simulink library "powerlib_modelsV2"  (Simulink 6.0)
settings: Solver=ode45  SolverMode=SingleTasking  StartTime=0.0  StopTime=10.0  RelTol=1e-3
undefined symbols (not defined in the file or in its folder): A, Ac, B, Bc, C, Cc, Cs, Current, damp, Dc, Dd, DiscIntNeverNeededParam, dref, dwo, exc, F, fb, gate, GH, GHd, GI, GId, GL, GLd, H, HT, hyd, ib, ib2, io, isfinite, j, K, Kd, Kg, L, Lad, Laq, lim, LIM, Ll, Llfd, Llkd, Llkq1, Llkq2, Llr, Lls, LowerFlux, N, N2, Nb, Nb2, nb_arm, p, Par_HarmoA_pu, Par_HarmoB_pu, Par_Timing_Harmo, Par_Timing_Variation, Par_Vps, Pb ... (+58)
libraries: powerlib_extras x14
(part 4 of 11)

== system powerlib_modelsV2/Continuous/simplified_sync_mach ==
  v : Inport  Port=1  LatchInput=off
  pm : Inport  Port=2  LatchInput=off
  e : Inport  Port=3  LatchInput=off
  1\p : Gain  Gain=1/p  SaturateOnIntegerOverflow=on
  Selector : Selector  Elements=sel  InputPortWidth=3
  Subsystem : Subsystem
  Vt : Subsystem
  Z : Subsystem
      mask Display: disp('Z')
  gen : Subsystem
      mask Display: disp('gen')
  ib : Gain  Gain=ib  SaturateOnIntegerOverflow=on
  mechanics : Subsystem
      mask Display: disp('mec')
  wattmeter : Subsystem  Orientation=left
      mask Display: disp('wattmeter')
  i : Outport  InitialOutput=0
  * : Outport  Port=2  InitialOutput=0
  wires:
  Selector/1 -> i/1
  ib/1 -> Selector/1
  wattmeter/1(Pe) -> mechanics/2(Pe), Subsystem/6(Pe)
  pm/1 -> mechanics/1(Pm)
  e/1 -> gen/2(E)
  mechanics/1(theta_e) -> 1\p/1, gen/1(theta)
  v/1 -> Vt/1(V)
  1\p/1 -> Subsystem/4(theta)
  mechanics/2(wm) -> Subsystem/5(wm)
  Z/1(i) -> ib/1, Subsystem/1(i), wattmeter/1(i)
  gen/1(e) -> Subsystem/3(e), Z/1(e), wattmeter/2(v)  "e"
  Vt/1(Vn) -> gen/3(Vn)
  Vt/2(Vabc) -> Z/2(v), Subsystem/2(v)
  Subsystem/1(*) -> */1

== system powerlib_modelsV2/Continuous/surge_arrester ==
  v : Inport  Port=1  LatchInput=off
  Abs : Abs  SaturateOnIntegerOverflow=on
  Break Alg. Loop : TransferFcn  Denominator="[0.01e-6  1]"
  Product : Product  SaturateOnIntegerOverflow=on  InputSameDT=on
  Sign : Signum  Orientation=down
  Switch1 : Switch  Threshold=ic1  InputSameDT=on
  Switch2 : Switch  Threshold=ic2  InputSameDT=on
  segment1 : Fcn  Expr=p1*(u/uref)^a1
  segment2 : Fcn  Expr=p2*(u/uref)^a2
  segment3 : Fcn  Expr=p3*(u/uref)^a3
  I : Outport  InitialOutput=0
  wires:
  Sign/1 -> Product/2
  Abs/1 -> segment1/1, segment2/1, segment3/1
  segment1/1 -> Switch1/3, Switch1/2
  segment2/1 -> Switch1/1
  Switch2/1 -> Product/1
  Switch1/1 -> Switch2/2, Switch2/3
  segment3/1 -> Switch2/1
  v/1 -> Break Alg. Loop/1
  Break Alg. Loop/1 -> Sign/1, Abs/1
  Product/1 -> I/1

== system powerlib_modelsV2/Continuous/synchronous_machine ==
  v : Inport  Port=1  PortDimensions=2  LatchInput=off
  pm : Inport  Port=2  PortDimensions=1  LatchInput=off
  vf : Inport  Port=3  PortDimensions=1  LatchInput=off
  Delta angle : Subsystem
  Mux : Mux  Inputs=[3,10,6,1,1,1]
  PQ : Subsystem
  Subsystem : Subsystem
  abc2qd : Subsystem
      mask Display: disp('abc/\nqd')
  currents and mutual fluxes : Subsystem
      mask Display: disp('currents\nand\nmutual\nfluxes')
  ia,ib : Selector  Elements=1:2  InputPortWidth=3
  mec : Subsystem
      mask Display: disp('mec')
  phid : Subsystem
      mask Display: disp('phid')
  phifd : Subsystem
      mask Display: disp('phifd')
  phikd : Subsystem
      mask Display: disp('phikd')
  phikq1 : Subsystem
      mask Display: disp('phikq1')
  phikq2 : Subsystem
      mask Display: disp('phikq2')
  phiq : Subsystem
      mask Display: disp('phiq')
  qd2abc : Subsystem
      mask Display: disp('qd/\nabc')
  vkd : Ground
  vkq2 : Ground
  i : Outport  InitialOutput=0
  m : Outport  Port=2  InitialOutput=0
  wires:
  vf/1 -> Subsystem/1(Vf)
  currents and mutual fluxes/2("iq,id,ifd, ikq1,ikq2,ikd, phimq,phimd,vq,vd") -> Mux/2
  vkq2/1 -> phikq2/1(vkq2)
  abc2qd/2(vq) -> phiq/1(vq), Delta angle/1(Vq), currents and mutual fluxes/7(vq), PQ/1(Vq)  "Vq"
  pm/1 -> mec/4(Pm)
  vkd/1 -> phikd/2(vkd)
  phiq/1(phiq) -> phid/2(phiq), mec/3(phiq), currents and mutual fluxes/1(phiq)
  qd2abc/1(is(A)) -> ia,ib/1  "iabc"
  currents and mutual fluxes/1(phimq) -> phiq/4(phimq), phikq2/2(phimq), phikq1/1(phimq)
  qd2abc/2(is(pu)) -> Mux/1
  abc2qd/1(cos,sin) -> qd2abc/1(sin,cos)  "sin,cos"
  currents and mutual fluxes/3(iq,id) -> qd2abc/2(iq,id), mec/1("iq,id "), PQ/3(Iq)  "iq,id"
  ia,ib/1 -> i/1
  phid/1(phid) -> currents and mutual fluxes/3(phid), phiq/3(phid), mec/2(phid)
  abc2qd/3(vd) -> phid/3(vd), Delta angle/2(Vd), currents and mutual fluxes/8(vd), PQ/2(Vd)  "Vd"
  v/1 -> abc2qd/1(v)
  phikd/1(phikd) -> currents and mutual fluxes/6(phikd)
  phifd/1(phifd) -> currents and mutual fluxes/4(phifd)
  phikq1/1(phikq1) -> currents and mutual fluxes/5(phikq1)
  phikq2/1(phikq2) -> currents and mutual fluxes/2(phikq2)
  Subsystem/1(Vkq1) -> phikq1/2(vkq1)
  Subsystem/2(Vfd) -> phifd/1(vfd)
  mec/2(thetae) -> abc2qd/2(theta)
  mec/3(we) -> phiq/2(w), phid/1(w)
  Mux/1 -> m/1
  mec/1(misc) -> Mux/3
  currents and mutual fluxes/4(phimd) -> phid/4(phimd), phifd/2(phimd), phikd/1(phimd)
  PQ/1(Peo) -> Mux/5
  PQ/2(Qeo) -> Mux/6
  Delta angle/1(delta) -> Mux/4

== system powerlib_modelsV2/Continuous/thyristor (logical) ==
  v : Inport  Port=1  LatchInput=off
  g : Inport  Port=2  LatchInput=off
  0 {1..4} (4 alike) : Constant  Value=0
  1/Rsw : Gain  Orientation=down  Gain=1./Rsw  SaturateOnIntegerOverflow=on
  Break Alg. Loop : Subsystem  mask{Nsw=1}
      mask prompts: Nsw "number of switches"
  Constant : Constant  Value=zeros(Nsw,1)
  Data Type  Conversion{1..4} (4 alike) : DataTypeConversion  SaturateOnIntegerOverflow=on  RndMeth=Zero
  Mux : Mux  Inputs=2
  Saturation : Saturate  UpperLimit=inf  LowerLimit=0
  Sum : Sum  Inputs=|++  SaturateOnIntegerOverflow=on  InputSameDT=on
  Switch : Switch  Threshold=0.5  InputSameDT=on
  b5 : RelationalOperator  Operator=>  InputSameDT=on
  b6 : RelationalOperator  Operator=>  InputSameDT=on
  b7 : RelationalOperator  Operator===  InputSameDT=on
  or2 : Logic  Operator=OR
  or3 : Logic  Inputs=3
  vf : Constant  Value=Vf
  i : Outport  InitialOutput=0
  Status : Outport  Port=2  InitialOutput=0
  m : Outport  Port=3  InitialOutput=0
  Vf : Outport  Port=4  InitialOutput=0
  wires:
  Data Type  Conversion4/1 -> or3/3
  Data Type  Conversion3/1 -> or3/2
  g/1 -> Data Type  Conversion4/1  "gate signal"
  0 2/1 -> b6/2
  or3/1 -> or2/2  "Gate = 1 Voltage > 0 Current = 0"
  Mux/1 -> m/1  "measurement signals"
  0 3/1 -> b7/2
  b7/1 -> Data Type  Conversion3/1  "Current = 0"
  or2/1 -> Break Alg. Loop/1(In1)
  Break Alg. Loop/1(Out1) -> Status/1, Switch/2
  0 1/1 -> b5/2
  Constant/1 -> i/1
  v/1 -> b6/1, Sum/1, 1/Rsw/1  "Vak"
  Sum/1 -> Mux/2
  vf/1 -> Sum/2, Vf/1
  b5/1 -> Data Type  Conversion1/1  "Current > 0"
  Data Type  Conversion1/1 -> or2/1
  b6/1 -> Data Type  Conversion2/1  "Voltage > 0"
  Data Type  Conversion2/1 -> or3/1
  Switch/1 -> Saturation/1
  0 4/1 -> Switch/3
  Saturation/1 -> Mux/1, b7/1, b5/1
  1/Rsw/1 -> Switch/1  "Iak"

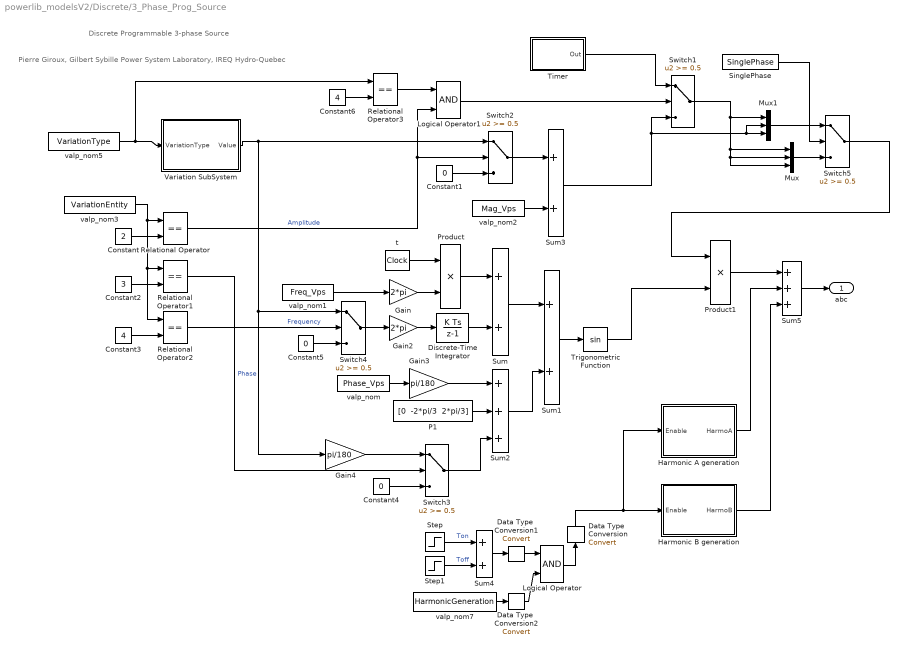
== system powerlib_modelsV2/Discrete/3_Phase_Prog_Source ==
  note: Pierre Giroux, Gilbert Sybille
      | Power System Laboratory, IREQ
      | Hydro-Quebec
  note: Discrete Programmable 3-phase Source
  Constant : Constant  Value=2
  Constant1 : Constant  Value=0
  Constant2 : Constant  Value=3
  Constant3 : Constant  Value=4
  Constant4 : Constant  Value=0
  Constant5 : Constant  Value=0
  Constant6 : Constant  Value=4
  Data Type  Conversion : DataTypeConversion  Orientation=up  SaturateOnIntegerOverflow=on  RndMeth=Zero
  Data Type  Conversion1 : DataTypeConversion  SaturateOnIntegerOverflow=on  RndMeth=Zero
  Data Type  Conversion2 : DataTypeConversion  SaturateOnIntegerOverflow=on  RndMeth=Zero
  Discrete-Time Integrator : DiscreteIntegrator  SampleTime=Ts  SaturateOnIntegerOverflow=on  ICPrevOutput=DiscIntNeverNeededParam  ICPrevScaledInput=DiscIntNeverNeededParam
  Gain : Gain  Gain=2*pi  SaturateOnIntegerOverflow=on
  Gain2 : Gain  Gain=2*pi  SaturateOnIntegerOverflow=on
  Gain3 : Gain  Gain=pi/180  SaturateOnIntegerOverflow=on
  Gain4 : Gain  Gain=pi/180  SaturateOnIntegerOverflow=on
  Harmonic A generation : Subsystem  mask(Harmonic generation){Freq_Vps=Freq_Vps, n_Harmo=n_HarmoA, Mag_Harmo=Mag_HarmoA, Phase_Harmo=Phase_HarmoA, Seq_Harmo=Seq_HarmoA, Ts=Ts}
      mask prompts: Ts "Sample time:"
  Harmonic B generation : Subsystem  mask(Harmonic generation){Freq_Vps=Freq_Vps, n_Harmo=n_HarmoB, Mag_Harmo=Mag_HarmoB, Phase_Harmo=Phase_HarmoB, Seq_Harmo=Seq_HarmoB, Ts=Ts}
      mask prompts: Ts "Sample time:"
  Logical Operator : Logic
  Logical Operator1 : Logic
  Mux : Mux  Inputs=3
  Mux1 : Mux  Inputs=3
  P1 : Constant  Value="[0  -2*pi/3  2*pi/3]"
  Product : Product  SaturateOnIntegerOverflow=on  InputSameDT=on
  Product1 : Product  SaturateOnIntegerOverflow=on  InputSameDT=on
  Relational Operator{,1..3} (4 alike) : RelationalOperator  Operator===  InputSameDT=on
  SinglePhase : Constant  Value=SinglePhase
  Step : Step  Time=Ton_Harmo  SampleTime=Ts
  Step1 : Step  Time=Toff_Harmo  After=-1  SampleTime=Ts
  Sum{,1,3..4} (4 alike) : Sum  SaturateOnIntegerOverflow=on  InputSameDT=on
  Sum2 : Sum  Inputs=+++  SaturateOnIntegerOverflow=on  InputSameDT=on
  Sum5 : Sum  Inputs=+++  SaturateOnIntegerOverflow=on  InputSameDT=on
  Switch{1..5} (5 alike) : Switch  Threshold=0.5  InputSameDT=on
  Timer : Subsystem  mask(Timer){t=Xtime, e=Yampli, Ts=Ts}
      mask prompts: t "Time (s):"; e "Amplitude:"; Ts "Sample time (s)"
      mask help:
      | Generates a signal changing  at specified times.
      |
      | Value of the signal at time zero must  be specified.
      mask init: same as powerlib_modelsV2/Continuous/3_Phase_Prog_Source/Timer
      mask Display: plot( tv(2:end-1), opv(2:end-1) )
  Trigonometric Function : Trigonometry
  Variation SubSystem : Subsystem  mask(Variation Subsystem){VariationStep=VariationStep, VariationRate=VariationRate, VariationFreq=VariationFreq, VariationMag=VariationMag, Ton_Variation=Ton_Variation, Toff_Variation=Toff_Variation, Ts=Ts}
      mask prompts: Ts "Sample time:"
  t : DigitalClock  SampleTime=Ts
  valp_nom : Constant  Value=Phase_Vps
  valp_nom1 : Constant  Value=Freq_Vps
  valp_nom2 : Constant  Value=Mag_Vps
  valp_nom3 : Constant  Value=VariationEntity
  valp_nom5 : Constant  Value=VariationType
  valp_nom7 : Constant  Value=HarmonicGeneration
  abc : Outport  InitialOutput=0
  wires:
  Logical Operator1/1 -> Switch1/2
  Relational Operator3/1 -> Logical Operator1/1
  Switch5/1 -> Product1/1
  Switch1/1 -> Mux1/1, Mux/3, Mux/2, Mux/1
  Mux/1 -> Switch5/3
  SinglePhase/1 -> Switch5/2
  Mux1/1 -> Switch5/1
  Timer/1(Out) -> Switch1/1
  Sum3/1 -> Mux1/2, Mux1/3, Switch1/3
  Constant6/1 -> Relational Operator3/2
  Gain4/1 -> Switch3/1
  Harmonic B generation/1(HarmoB) -> Sum5/3
  Step1/1 -> Sum4/2  "Toff"
  Step/1 -> Sum4/1  "Ton"
  Sum5/1 -> abc/1
  Harmonic A generation/1(HarmoA) -> Sum5/2
  Constant5/1 -> Switch4/3
  Constant3/1 -> Relational Operator2/2
  Constant2/1 -> Relational Operator1/2
  valp_nom3/1 -> Relational Operator1/1, Relational Operator2/1, Relational Operator/1
  Constant/1 -> Relational Operator/2
  Relational Operator2/1 -> Switch4/2  "Frequency"
  Switch4/1 -> Gain2/1
  Variation SubSystem/1(Value) -> Gain4/1, Switch4/1, Switch2/1
  Relational Operator1/1 -> Switch3/2  "Phase"
  Constant4/1 -> Switch3/3
  Switch3/1 -> Sum2/3
  valp_nom5/1 -> Relational Operator3/1, Variation SubSystem/1(VariationType)
  Relational Operator/1 -> Logical Operator1/2, Switch2/2  "Amplitude"
  valp_nom2/1 -> Sum3/2
  Sum2/1 -> Sum1/2
  Constant1/1 -> Switch2/3
  Switch2/1 -> Sum3/1
  Product1/1 -> Sum5/1
  valp_nom1/1 -> Gain/1
  valp_nom/1 -> Gain3/1
  Gain3/1 -> Sum2/1
  Trigonometric Function/1 -> Product1/2
  P1/1 -> Sum2/2
  Discrete-Time Integrator/1 -> Sum/2
  Gain2/1 -> Discrete-Time Integrator/1
  Sum1/1 -> Trigonometric Function/1
  Sum/1 -> Sum1/1
  t/1 -> Product/1
  Gain/1 -> Product/2
  Product/1 -> Sum/1
  Logical Operator/1 -> Data Type  Conversion/1
  Data Type  Conversion/1 -> Harmonic A generation/1(Enable), Harmonic B generation/1(Enable)
  Sum4/1 -> Data Type  Conversion1/1
  Data Type  Conversion1/1 -> Logical Operator/1
  valp_nom7/1 -> Data Type  Conversion2/1
  Data Type  Conversion2/1 -> Logical Operator/2

== system powerlib_modelsV2/Discrete/3_phase_source ==
  Constant : Constant  Value=complex(A*cos(P*pi/180),A*sin(P*pi/180))
  Constant1 : Constant  Value=complex(A*cos((P-120)*pi/180),A*sin((P-120)*pi/180))
  Constant2 : Constant  Value=complex(A*cos((P+120)*pi/180),A*sin((P+120)*pi/180))
  Mux : Mux  Inputs=6
  Sine Wave : Sin  Amplitude=A  Frequency=2*pi*F  Phase=P*pi/180  SampleTime=Ts
  Sine Wave1 : Sin  Amplitude=A  Frequency=2*pi*F  Phase=(P-120)*pi/180  SampleTime=Ts
  Sine Wave2 : Sin  Amplitude=A  Frequency=2*pi*F  Phase=(P+120)*pi/180  SampleTime=Ts
  Out1 : Outport
  wires:
  Mux/1 -> Out1/1
  Constant2/1 -> Mux/6
  Sine Wave2/1 -> Mux/5
  Constant1/1 -> Mux/4
  Sine Wave1/1 -> Mux/3
  Sine Wave/1 -> Mux/1
  Constant/1 -> Mux/2

== system powerlib_modelsV2/Discrete/Dynamic_Load ==
  v : Inport  Port=1  PortDimensions=2  LatchInput=off
  PQ : Inport  Port=2  PortDimensions=2  LatchInput=off
  Complex to Real-Imag : ComplexToRealImag  Orientation=left
  Demux : Demux  Outputs=2
  Discrete 3-phase PLL : Subsystem  mask(Discrete 3-phase PLL){Par_Init=[Pha_V0  fnom], ParK=[60 1400], Ts=Ts}
      mask prompts: Par_Init "Initial inputs:[ Phase(degrees)   Frequency(Hz) ]"; ParK "Regulator gains [ Kp  Ki ]"; Ts "Sample time:"
      mask init:
      | Kp=ParK(1);
      | Ki=ParK(2);
      | Phase_Init=Par_Init(1);
      | Finit=Par_Init(2);
  Discrete Variable Frequency Mean value : powerlib_extras/Discrete Measurements/Discrete Variable Frequency Mean value  Finit=fnom  Fmin=45  Vinit=Mag_V0  Ts=Ts
  Discrete Variable Frequency Mean value1 : powerlib_extras/Discrete Measurements/Discrete Variable Frequency Mean value  Finit=fnom  Fmin=45  Vinit=0  Ts=Ts
  Ground : Ground  Orientation=left
  Mux1 : Mux  Orientation=left  Inputs=3
  Positive Sequence  current : Subsystem
  Real-Imag to Complex : RealImagToComplex
  Real-Imag to Complex1 : RealImagToComplex
  Selector : Selector  Orientation=left  Elements=1:2  InputPortWidth=3
  Unit Delay2 : UnitDelay  Orientation=left  X0=I1_init*exp(-j*Pha_V0*pi/180)  SampleTime=Ts
  V> pu : Gain  Gain=1/Vbase  SaturateOnIntegerOverflow=on
  dq0_to_abc Transformation : powerlib_extras/Measurements/dq0_to_abc Transformation  Orientation=left
  i : Outport  Orientation=left
  m : Outport  Port=2
  wires:
  dq0_to_abc Transformation/1 -> Selector/1
  Selector/1 -> i/1
  v/1 -> V> pu/1
  V> pu/1 -> Discrete 3-phase PLL/1(Vab_bc (pu))
  Real-Imag to Complex/1 -> Positive Sequence  current/1(V1(pu))
  Mux1/1 -> dq0_to_abc Transformation/1
  Unit Delay2/1 -> Complex to Real-Imag/1
  Discrete 3-phase PLL/3(Vq) -> Discrete Variable Frequency Mean value1/2
  Ground/1 -> Mux1/3
  Discrete Variable Frequency Mean value/1 -> Real-Imag to Complex/1
  Discrete Variable Frequency Mean value1/1 -> Real-Imag to Complex/2
  Positive Sequence  current/1(I1(A)) -> Unit Delay2/1
  Complex to Real-Imag/1 -> Mux1/1
  Complex to Real-Imag/2 -> Mux1/2
  Discrete 3-phase PLL/2(Vd) -> Discrete Variable Frequency Mean value/2
  Discrete 3-phase PLL/4(sin_cos) -> dq0_to_abc Transformation/2
  Discrete 3-phase PLL/1(Freq) -> Discrete Variable Frequency Mean value/1, Discrete Variable Frequency Mean value1/1
  PQ/1 -> Demux/1
  Demux/1 -> Real-Imag to Complex1/1
  Demux/2 -> Real-Imag to Complex1/2
  Real-Imag to Complex1/1 -> Positive Sequence  current/2(S_ext)
  Positive Sequence  current/2(VPQ) -> m/1

== system powerlib_modelsV2/Discrete/Excitation_System ==
  vref : Inport  Port=1  LatchInput=off
  vd : Inport  Port=2  LatchInput=off
  vq : Inport  Port=3  LatchInput=off
  vstab : Inport  Port=4  LatchInput=off
  Damping kf.s / (tf.s +1) : Subsystem  Orientation=left
  Exciter  1 / (te.s + ke) : Subsystem
  Lead Lag Compensator tc.s+1 / tb.s+1 : powerlib_extras/Discrete  Control Blocks/Discrete Lead-Lag  T1=tc  T2=tb  V_Init=ke*v0(2)/ka  Ts=Ts
  Low Pass Filter 1 / (tr.s +1) (with IC) : powerlib_extras/Discrete  Control Blocks/Discrete 1st-Order Discrete Filter  FilterType=Lowpass  Tc=tr  Ts=Ts  Initialize=on  Vac_Init=[0 0 60]  Vdc_Init=v0(1)  PlotResponse=off  param1=[1 500 0.1]
  Main Regulator ka / (ta.s +1) : Subsystem
  Mux : Mux  Inputs=2
  Positive Seqence Voltage : Fcn  Expr=sqrt(u(1)^2 + u(2)^2)
  Sum : Sum  Inputs=++-+-  SaturateOnIntegerOverflow=on  InputSameDT=on
  Unit Delay1 : UnitDelay  Orientation=left  SampleTime=Ts
  Unit Delay2 : UnitDelay  X0=v0(2)  SampleTime=Ts
  Vf0 \ ka : Constant  Value=v0(2)/ka
  proportionnal saturation : Subsystem
  Vf : Outport  InitialOutput=0
  wires:
  Unit Delay2/1 -> Vf/1
  Unit Delay1/1 -> Sum/5
  proportionnal saturation/1(Ef) -> Exciter  1 / (te.s + ke)/1(In)
  Lead Lag Compensator tc.s+1 / tb.s+1/1 -> Main Regulator ka / (ta.s +1)/1(In)
  Sum/1 -> Lead Lag Compensator tc.s+1 / tb.s+1/1
  Positive Seqence Voltage/1 -> Low Pass Filter 1 / (tr.s +1) (with IC)/1
  vq/1 -> Mux/2
  vd/1 -> Mux/1
  Mux/1 -> Positive Seqence Voltage/1
  vref/1 -> Sum/1
  vstab/1 -> Sum/4
  Low Pass Filter 1 / (tr.s +1) (with IC)/1 -> proportionnal saturation/2(Vtf), Sum/3
  Vf0 \ ka/1 -> Sum/2
  Main Regulator ka / (ta.s +1)/1(Out) -> proportionnal saturation/1(Efd)
  Damping kf.s / (tf.s +1)/1(Out) -> Unit Delay1/1
  Exciter  1 / (te.s + ke)/1(Out) -> Unit Delay2/1, Damping kf.s / (tf.s +1)/1(In)

== system powerlib_modelsV2/Discrete/GTO-IGBT Bridge ==
  note: *
      | *
      | ||
      | ||
      | *
      | *
      | *
      | ||
      | ||
      | *
      | *
  note: 1
  note: 2
  note: +
  note: -
  note: *
      | *
      | ||
      | ||
      | *
      | *
      | *
      | ||
      | ||
      | *
      | *
  note: 3
  note: 4
  note: ***********************************************
  note: Vcc
  note: A
  note: B
  note: *
      | *
      | ||
      | ||
      | *
      | *
      | *
      | ||
      | ||
      | *
      | *
  note: C
  note: ***********************************************
  note: 5
  note: 6
  note: GTO:
      |  tail current can be turned off by specifying Tf=0 and Tt=0
  note: Diode Logic :
      | 1) Diodes are blocked when complementary GTOs are switched on
      | 2) When no snubber capacitances are used (Cs=inf), diodes are triggered
      | when complementary GTOs are swithed off
  v : Inport  Port=1  LatchInput=off
  g : Inport  Port=2  LatchInput=off
  1/Rsw : Gain  Orientation=up  Gain=1./Rsw  SaturateOnIntegerOverflow=on
  2 : Constant  Value=Tf>0 | Tt>0
  Constant1 : Constant  Value=0
  Data Type  Conversion{2..5} (4 alike) : DataTypeConversion  SaturateOnIntegerOverflow=on  RndMeth=Zero
  Diode Logic : Subsystem
  GTO Logic : Subsystem
  G_D : Logic  Operator=OR
  Gain : Gain  Orientation=up  Gain=-1  SaturateOnIntegerOverflow=on
  Product : Product  SaturateOnIntegerOverflow=on  InputSameDT=on
  Relational Operator : RelationalOperator  InputSameDT=on
  Tail discrete : Subsystem  TreatAsAtomicUnit=on  mask(Gto tail current){}
  Unit Delay : UnitDelay  SampleTime=Ts
  Unit Delay3 : UnitDelay  SampleTime=Ts
  "Vf " : Subsystem
  iTail : Outport
  status : Outport  Port=2
  Vf : Outport  Port=3
  wires:
  2/1 -> Tail discrete/Enable
  Relational Operator/1 -> Diode Logic/2(Ipos), Data Type  Conversion3/1
  Constant1/1 -> Relational Operator/2
  Unit Delay/1 -> Tail discrete/1(Iak)
  Gain/1 -> Diode Logic/1(Vak)
  Product/1 -> Unit Delay/1  "IGTO"
  Tail discrete/1(itail) -> iTail/1
  1/Rsw/1 -> Product/2, Relational Operator/1
  v/1 -> Gain/1, GTO Logic/1(Vak), 1/Rsw/1
  "Vf "/1(Vf) -> Vf/1
  GTO Logic/1(status) -> G_D/2, Diode Logic/3(G), "Vf "/1(status_GTO)
  Data Type  Conversion3/1 -> Product/1
  g/1 -> Data Type  Conversion4/1
  Data Type  Conversion4/1 -> Tail discrete/2(switch), GTO Logic/2(G)
  Diode Logic/1(status) -> Data Type  Conversion5/1
  Data Type  Conversion5/1 -> G_D/1
  Unit Delay3/1 -> status/1
  G_D/1 -> Data Type  Conversion2/1
  Data Type  Conversion2/1 -> Unit Delay3/1

== system powerlib_modelsV2/Discrete/HTG ==
  wref : Inport  Port=1  LatchInput=off
  Pref : Inport  Port=2  LatchInput=off
  we : Inport  Port=3  LatchInput=off
  Pe : Inport  Port=4  LatchInput=off
  dw : Inport  Port=5  LatchInput=off
  Constant1 : Constant  Orientation=left  Value=dref
  Discrete PID Controller : Subsystem  AncestorBlock=|  mask(Discrete PID Controller){Kp=kp, Ki=ki, Kd=kd, TcD=td, Par_Limits=[1e6 -1e6], Init=go, Ts=Ts}
      | powerlib_extras/Discrete 
      | Control Blocks/Discrete
      | PID Controller
      mask prompts: Kp "Proportional gain (Kp):"; Ki "Integral gain (Ki):"; Kd "Derivative gain (Kd):"; TcD "Time constant for derivative (s):"; Par_Limits "Output limits: [ Upper   Lower ]"; Init "Output initial value:"; Ts "Sample time:"
      mask help: This block implements a discrete PID controller.
      mask init:
      | UpperLimit=Par_Limits(1);
      | LowerLimit=Par_Limits(2);
      mask Display: disp('PID');
  Sum : Sum  Inputs=+-  SaturateOnIntegerOverflow=on  InputSameDT=on
  Sum1 : Sum  Inputs=+-  SaturateOnIntegerOverflow=on  InputSameDT=on
  Sum5 : Sum  Inputs=-+  SaturateOnIntegerOverflow=on  InputSameDT=on
  Switch : Switch  Orientation=left  Threshold=0.5  InputSameDT=on
  permanent droop : Gain  Orientation=left  Gain=Rp  SaturateOnIntegerOverflow=on
  servo-motor : Subsystem
      mask Display: disp('servo-\nmotor')
  turbine : Subsystem
      mask Display: disp('hydraulic\nturbine')
  Pm : Outport  InitialOutput=0
  gate : Outport  Port=2  InitialOutput=0
  wires:
  Constant1/1 -> Switch/2
  Switch/1 -> permanent droop/1
  Pe/1 -> Sum5/2
  Pref/1 -> Sum5/1
  Sum1/1 -> Discrete PID Controller/1(Error)
  permanent droop/1 -> Sum1/2
  Sum/1 -> Sum1/1
  Discrete PID Controller/1(Out) -> servo-motor/1(regulator's output)
  wref/1 -> Sum/1
  we/1 -> Sum/2
  Sum5/1 -> Switch/3
  servo-motor/1(gate opening) -> turbine/2(gate opening), gate/1, Switch/1
  dw/1 -> turbine/1(dw)
  turbine/1(Pm) -> Pm/1

== system powerlib_modelsV2/Discrete/Impedance Measurement ==
  v : Inport  Port=1  LatchInput=off
  Ground : Ground
  Terminator : Terminator
  i : Outport  InitialOutput=0
  wires:
  v/1 -> Terminator/1
  Ground/1 -> i/1

== system powerlib_modelsV2/Discrete/MBPSS ==
  note: (for simplified
      | settings only)
  note: Low and intermediate speed deviation is based on the internal voltage phasors while
      | the high frequency speed deviation  is based on the electrical power.
  note: Note: Speed deviation is derived from the machine positive-sequence terminal voltages and currents.
  note: (IEEE Type PSS4b)
  note: Discrete Multi-band Power System Stabilizer
  note: Innocent Kamwa, Robert Grondin
      | IREQ, Hydro-Quebec
  dw : Inport  Port=1  LatchInput=off
  Constant : Constant  Value=Detailed
  Discrete Lead-Lag1 : Subsystem  mask(Discrete Lead-Lag Compensator){values=[TL1 TL2 KL11], Ts=Ts}
      mask prompts: values "Coefficients values: [ T1 T2 K1 ]"; Ts "Sample time (s):"
      mask help:
      | This block implements a discrete lead-lag compensator:
      |
      |          T1.s + K1
      | H(s)= --------
      |            T2.s + 1
      mask init:
      | numc=[values(1) values(3)];
      | denc=[values(2) 1];
      | [Ac,Bc,Cc,Dc]=tf2ss(numc,denc);
      | %
      | %  Conversion to discrete transfer function
      | nstates = size(Ac,1);
      | invexp = inv(eye(nstates) - (Ts/2)*Ac);
      | Ad = invexp*(eye(nstates) + (Ts/2)*Ac);
      | Bd = invexp*Bc;
      | Cd = Cc*invexp*Ts;
      | Dd = Cc*invexp*Bc*(Ts/2) + Dc;
      | %
      | if values(1)==0 & values(2)==0, Dd=1; end
      mask Display: disp('TL1.s+KL11\n---\nTL2.s+1')
  Discrete Lead-Lag2 : Subsystem  mask(Discrete Lead-Lag Compensator){values=[TL7 TL8 KL17], Ts=Ts}
      mask prompts: values "Coefficients values: [ T1 T2 K1 ]"; Ts "Sample time (s):"
      mask help:
      | This block implements a discrete lead-lag compensator:
      |
      |          T1.s + K1
      | H(s)= --------
      |            T2.s + 1
      mask init: same as powerlib_modelsV2/Discrete/MBPSS/Discrete Lead-Lag1
      mask Display: disp('TL7.s+KL17\n---\nTL8.s+1')
  Discrete Lead-Lag3 : Subsystem  mask(Discrete Lead-Lag Compensator){values=[TI1 TI2 KI11], Ts=Ts}
      mask prompts: values "Coefficients values: [ T1 T2 K1 ]"; Ts "Sample time (s):"
      mask help:
      | This block implements a discrete lead-lag compensator:
      |
      |          T1.s + K1
      | H(s)= --------
      |            T2.s + 1
      mask init: same as powerlib_modelsV2/Discrete/MBPSS/Discrete Lead-Lag1
      mask Display: disp('TI1.s+KI11\n---\nTI2.s+1')
  Discrete Lead-Lag4 : Subsystem  mask(Discrete Lead-Lag Compensator){values=[TI7 TI8 KI17], Ts=Ts}
      mask prompts: values "Coefficients values: [ T1 T2 K1 ]"; Ts "Sample time (s):"
      mask help:
      | This block implements a discrete lead-lag compensator:
      |
      |          T1.s + K1
      | H(s)= --------
      |            T2.s + 1
      mask init: same as powerlib_modelsV2/Discrete/MBPSS/Discrete Lead-Lag1
      mask Display: disp('TI7.s+KI17\n---\nTI8.s+1')
  Discrete Lead-Lag5 : Subsystem  mask(Discrete Lead-Lag Compensator){values=[TH1 TH2 KH11], Ts=Ts}
      mask prompts: values "Coefficients values: [ T1 T2 K1 ]"; Ts "Sample time (s):"
      mask help:
      | This block implements a discrete lead-lag compensator:
      |
      |          T1.s + K1
      | H(s)= --------
      |            T2.s + 1
      mask init: same as powerlib_modelsV2/Discrete/MBPSS/Discrete Lead-Lag1
      mask Display: disp('TH1.s+KH11\n---\nTH2.s+1')
  Discrete Lead-Lag6 : Subsystem  mask(Discrete Lead-Lag Compensator){values=[TH7 TH8 KH17], Ts=Ts}
      mask prompts: values "Coefficients values: [ T1 T2 K1 ]"; Ts "Sample time (s):"
      mask help:
      | This block implements a discrete lead-lag compensator:
      |
      |          T1.s + K1
      | H(s)= --------
      |            T2.s + 1
      mask init: same as powerlib_modelsV2/Discrete/MBPSS/Discrete Lead-Lag1
      mask Display: disp('TH7.s+KH17\n---\nTH8.s+1')
  Gain : Gain  Gain=KL  SaturateOnIntegerOverflow=on
  Gain1 : Gain  Gain=KI  SaturateOnIntegerOverflow=on
  Gain2 : Gain  Gain=KH  SaturateOnIntegerOverflow=on
  Gain3 : Gain  Gain=KL1  SaturateOnIntegerOverflow=on
  Gain4 : Gain  Gain=KL2  SaturateOnIntegerOverflow=on
  Gain5 : Gain  Gain=KI1  SaturateOnIntegerOverflow=on
  Gain6 : Gain  Gain=KI2  SaturateOnIntegerOverflow=on
  Gain7 : Gain  Gain=KH1  SaturateOnIntegerOverflow=on
  Gain8 : Gain  Gain=KH2  SaturateOnIntegerOverflow=on
  Gain9 : Gain  Gain=Kg  SaturateOnIntegerOverflow=on
  HF speed sensor : Subsystem  mask(discrete state-space model (PSB)){numc=[80 0 0], denc=[1 82 161 80], Ts=Ts}
      mask prompts: numc "Numerator:"; denc "Denominator:"; Ts "Sample time (s):"
      mask help: This block implements a discrete state-space model based on the coefficients of a continuous transfer function. Coefficients must be given in descending power of s.
      mask init:
      | [Ac,Bc,Cc,Dc]=tf2ss(numc,denc);
      | %
      | %  Conversion to discrete transfer function
      | nstates = size(Ac,1);
      | invexp = inv(eye(nstates) - (Ts/2)*Ac);
      | Ad = invexp*(eye(nstates) + (Ts/2)*Ac);
      | Bd = invexp*Bc;
      | Cd = Cc*invexp*Ts;
      | Dd = Cc*invexp*Bc*(Ts/2) + Dc;
      mask Display: disp('Discrete\nState-space\nModel')
  LF and IF speed sensor : Subsystem  mask(discrete state-space model (PSB)){numc=[-1.759e-3 1], denc=[1.2739e-4 1.7823e-2 1], Ts=Ts}
      mask prompts: numc "Numerator:"; denc "Denominator:"; Ts "Sample time (s):"
      mask help: This block implements a discrete state-space model based on the coefficients of a continuous transfer function. Coefficients must be given in descending power of s.
      mask init: same as powerlib_modelsV2/Discrete/MBPSS/HF speed sensor
      mask Display: disp('Discrete\nState-space\nModel')
  "Limiteur BF " : Saturate  UpperLimit=LIM_VL  LowerLimit=-LIM_VL
  Limiteur HF : Saturate  UpperLimit=LIM_VH  LowerLimit=-LIM_VH
  "Limiteur IF " : Saturate  UpperLimit=LIM_VI  LowerLimit=-LIM_VI
  Limiteur VS : Saturate  UpperLimit=LIM_VS  LowerLimit=-LIM_VS
  Sum : Sum  Inputs=+-  SaturateOnIntegerOverflow=on  InputSameDT=on
  Sum1 : Sum  Inputs=+++  SaturateOnIntegerOverflow=on  InputSameDT=on
  Sum2 : Sum  Inputs=+-  SaturateOnIntegerOverflow=on  InputSameDT=on
  Sum3 : Sum  Inputs=+-  SaturateOnIntegerOverflow=on  InputSameDT=on
  Transfer function for detailed model (HF) : Subsystem
  Transfer function for detailed model (IF) : Subsystem
  Transfer function for detailed model (LF) : Subsystem
  VS : Outport  InitialOutput=0
  wires:
  Gain9/1 -> Limiteur VS/1
  Constant/1 -> Transfer function for detailed model (HF)/1(On), Transfer function for detailed model (IF)/1(On), Transfer function for detailed model (LF)/1(On)
  Limiteur VS/1 -> VS/1
  Sum1/1 -> Gain9/1
  Limiteur HF/1 -> Sum1/3
  "Limiteur IF "/1 -> Sum1/2
  "Limiteur BF "/1 -> Sum1/1
  Sum3/1 -> Gain2/1
  Transfer function for detailed model (HF)/2(LFneg) -> Sum3/2
  Transfer function for detailed model (HF)/1(HFpos) -> Sum3/1
  Discrete Lead-Lag6/1(Out1) -> Transfer function for detailed model (HF)/3("HFneg ")
  Discrete Lead-Lag5/1(Out1) -> Transfer function for detailed model (HF)/2("HFpos ")
  Sum2/1 -> Gain1/1
  Discrete Lead-Lag4/1(Out1) -> Transfer function for detailed model (IF)/3("IFneg ")
  Discrete Lead-Lag3/1(Out1) -> Transfer function for detailed model (IF)/2("IFpos ")
  Transfer function for detailed model (IF)/2(IFneg) -> Sum2/2
  Transfer function for detailed model (IF)/1(IFpos) -> Sum2/1
  Discrete Lead-Lag2/1(Out1) -> Transfer function for detailed model (LF)/3("LFneg ")
  Discrete Lead-Lag1/1(Out1) -> Transfer function for detailed model (LF)/2("LFpos ")
  Transfer function for detailed model (LF)/2(LFneg) -> Sum/2
  Transfer function for detailed model (LF)/1(LFpos) -> Sum/1
  Sum/1 -> Gain/1
  Gain/1 -> "Limiteur BF "/1
  Gain1/1 -> "Limiteur IF "/1
  Gain2/1 -> Limiteur HF/1
  Gain3/1 -> Discrete Lead-Lag1/1(In1)
  Gain4/1 -> Discrete Lead-Lag2/1(In1)
  Gain5/1 -> Discrete Lead-Lag3/1(In1)
  Gain6/1 -> Discrete Lead-Lag4/1(In1)
  Gain7/1 -> Discrete Lead-Lag5/1(In1)
  Gain8/1 -> Discrete Lead-Lag6/1(In1)
  LF and IF speed sensor/1(Out) -> Gain3/1, Gain4/1, Gain5/1, Gain6/1
  HF speed sensor/1(Out) -> Gain8/1, Gain7/1
  dw/1 -> HF speed sensor/1(In), LF and IF speed sensor/1(In)

== system powerlib_modelsV2/Discrete/PM_synchronous_machine ==
  v : Inport  Port=1  LatchInput=off
  Tm : Inport  Port=2  LatchInput=off
  Mux : Mux  Inputs=[3,2,2,3]
  Selector : Selector  Elements=1:2  InputPortWidth=3
  abc2qd : Subsystem
  iq,id : Subsystem
  mec : Subsystem  Orientation=left
  qd2abc : Subsystem
  i : Outport  InitialOutput=0
  m : Outport  Port=2  InitialOutput=0
  wires:
  mec/2(the) -> abc2qd/2(the)
  mec/3(w,th,Te) -> Mux/4  "w,th,Te"
  Tm/1 -> mec/1(Tm)
  mec/1(we) -> iq,id/2(we)
  Mux/1 -> m/1
  abc2qd/2(vq,vd) -> Mux/3, iq,id/1(vq,vd)  "vqd"
  abc2qd/1(s,c) -> qd2abc/1(s,c)
  v/1 -> abc2qd/1(Vab,Vbc)
  iq,id/1(iq,id) -> Mux/2, mec/2(iq,id), qd2abc/2(iq,id)  "iqd"
  qd2abc/1(is) -> Mux/1, Selector/1  "isabc"
  Selector/1 -> i/1

== system powerlib_modelsV2/Discrete/PSS ==
  note: Power System Stabilizer (PSS)
      | (Discrete generic model)
  In : Inport  Port=1  LatchInput=off
  Lead-Lag #1 : Subsystem  AncestorBlock=|  mask(Discrete Lead-Lag Controller){T1=T1n, T2=T1d, V_Init=0, Ts=Ts}
      | powerlib_extras/Discrete 
      | Control Blocks/Discrete
      | Lead-Lag
      mask prompts: T1 "Time constant T1 (s):"; T2 "Time constant T2 (s):"; V_Init "Initial input and output:"; Ts "Sample time (s):"
      mask help:
      | This block implements a discrete lead-lag controller:
      |
      |          1+T1s
      | H(s)= ------
      |          1+T2s
      |
      | States are initialized according to initial input anf output value so that simulation starts in steady state.
      mask init:
      | numc=[T1 1];
      | denc=[T2 1];
      | [Ac,Bc,Cc,Dc]=tf2ss(numc,denc);
      | 
      | %  Conversion to discrete transfer function
      | nstates = size(Ac,1);
      | invexp = inv(eye(nstates) - (Ts/2)*Ac);
      | Ad = invexp*(eye(nstates) + (Ts/2)*Ac);
      | Bd = invexp*Bc;
      | Cd = Cc*invexp*Ts;
      | Dd = Cc*invexp*Bc*(Ts/2) + Dc;
      | %
      | % Compute Initial states
      | I=eye(size(Ac));
      | x0c=inv(-Ac)*Bc*V_Init;
      | x0d=(I-Ac*Ts/2)*x0c/Ts - Bc/2*V_Init;
      | 
      | if T1==0 & T2==0, Dd=1; end
      mask Display: disp('1+T1s\n---\n1+T2s')
  Lead-Lag #2 : Subsystem  AncestorBlock=|  mask(Discrete Lead-Lag Controller){T1=T2n, T2=T2d, V_Init=0, Ts=Ts}
      | powerlib_extras/Discrete 
      | Control Blocks/Discrete
      | Lead-Lag
      mask prompts: T1 "Time constant T1 (s):"; T2 "Time constant T2 (s):"; V_Init "Initial input and output:"; Ts "Sample time (s):"
      mask help:
      | This block implements a discrete lead-lag controller:
      |
      |          1+T1s
      | H(s)= ------
      |          1+T2s
      |
      | States are initialized according to initial input anf output value so that simulation starts in steady state.
      mask init: same as powerlib_modelsV2/Discrete/PSS/Lead-Lag #1
      mask Display: disp('1+T1s\n---\n1+T2s')
  "Limiter " : Saturate  UpperLimit=VSlimits(2)  LowerLimit=VSlimits(1)
  Overall Gain : Gain  Gain=K  SaturateOnIntegerOverflow=on
  "Sensor " : Subsystem  AncestorBlock=|  mask(Discrete 1st-Order Filter){FilterType=Lowpass, Tc=Tsensor, Ts=Ts, Initialize=on, Vac_Init=[0 0 60], Vdc_Init=Vinit, PlotResponse=off, param1=[1 500 0.1]}
      | powerlib_extras/Discrete 
      | Control Blocks/Discrete
      | 1st-Order
      | Discrete Filter
      mask prompts: FilterType "Filter Type:"; Tc "Time constant (s):"; Ts "Sample time:"; Initialize "Initialize filter states"; Vac_Init "AC initial input: [ Mag  Phase(degrees)  Freq(Hz) ]"; Vdc_Init "DC Initial input:"; PlotResponse "Plot filter response"; param1 "Frequency range(Hz) : [Start  End  Inc.]"
      mask init:
      | switch FilterType
      | case 1, % Lowpass
      |        X=[0 1 2 3 4];
      |        Y=[-2 -2 -3 -4 -4];
      |        numc=1;
      |        denc=[Tc 1];
      |  case 2,   % Highpass
      |        X=[0 1 2 3 4];
      |        Y=[-4 -4 -3 -2 -2];
      |         numc=[1 0];
      |         denc=[1 1/Tc];
      | end
      | %
      | [Ac,Bc,Cc,Dc]=tf2ss(numc,denc);
      | %
      | %  Conversion to discrete transfer function
      | nstates = size(Ac,1);
      | invexp = inv(eye(nstates) - (Ts/2)*Ac);
      | Ad = invexp*(eye(nstates) + (Ts/2)*Ac);
      | Bd = invexp*Bc;
      | Cd = Cc*invexp*Ts;
      | Dd = Cc*invexp*Bc*(Ts/2) + Dc;
      | %
      | if Initialize==1  % Compute initial conditions on states
      | u1=Vac_Init(1)*exp(j*Vac_Init(2)*pi/180);
      | u2=Vdc_Init*exp(j*90*pi/180);
      | u=u1+u2;
      | u0=imag(u); % input at  t=0;
      | I=eye(size(Ac));
      | sI1=I*j*(2*pi*Vac_Init(3));
      | sI2=I*j*0;
      | x=inv(sI1-Ac)*Bc*u1 + inv(sI2-Ac)*Bc*u2;
      | x0c=imag(x);
      | x0d=(I-Ac*Ts/2)*x0c/Ts - Bc/2*u0;
      | else
      | x0d=0;
      | end
      | 
      | %
      | if PlotResponse==1 % Plot frequency and step response
      | figure(1)
      | sys=ss(Ad,Bd,Cd,Dd,Ts);
      | f=param1(1):param1(3):param1(2);
      | w=2*pi*f;
      | [mag phase]=bode(sys,w);
      | subplot(2,1,1)
      | plot(f,squeeze(mag))
      | title('Magnitude')
      | grid
      | subplot(2,1,2)
      | plot(f,squeeze(phase))
      | title('Phase (degrees)')
      | xlabel('Hz')
      | grid
      | figure(2)
      | step(sys)
      | end
      mask StyleString: popup(Lowpass|Highpass),edit,edit,checkbox,edit,edit,checkbox,edit
      mask CallbackString: |||p4=get_param(gcb,'Initialize');if strcmp(p4,'on');visible={'on','on','on','on','on','on','on',get_param(gcb,'PlotResponse')};else;visible={'on','on','on','on','off','off','on',get_param(gcb,'PlotResponse')};end;set_param(gcb,'MaskVisibilities',visible)|||p7=get_param(gcb,'PlotResponse');if strcmp(p7,'on');visible={'on','on','on','on',get_param(gcb,'Initialize'),get_param(gcb,'Initialize'),'on','on'};else;visible={'on','on','on','on',get_param(gcb,'Initialize'),get_param(gcb,'Initialize'),'on','off'};end;set_param(gcb,'MaskVisibilities',visible)|
      mask Display: plot(X,Y);
  "Wash-out " : Subsystem  AncestorBlock=|  mask(Discrete 1st-Order Filter){FilterType=Highpass, Tc=Twashout, Ts=Ts, Initialize=on, Vac_Init=[0 0 60], Vdc_Init=K*Vinit, PlotResponse=off, param1=[1 500 0.1]}
      | powerlib_extras/Discrete 
      | Control Blocks/Discrete
      | 1st-Order
      | Discrete Filter
      mask prompts: FilterType "Filter Type:"; Tc "Time constant (s):"; Ts "Sample time:"; Initialize "Initialize filter states"; Vac_Init "AC initial input: [ Mag  Phase(degrees)  Freq(Hz) ]"; Vdc_Init "DC Initial input:"; PlotResponse "Plot filter response"; param1 "Frequency range(Hz) : [Start  End  Inc.]"
      mask init: same as powerlib_modelsV2/Discrete/PSS/Sensor 
      mask StyleString: popup(Lowpass|Highpass),edit,edit,checkbox,edit,edit,checkbox,edit
      mask CallbackString: |||p4=get_param(gcb,'Initialize');if strcmp(p4,'on');visible={'on','on','on','on','on','on','on',get_param(gcb,'PlotResponse')};else;visible={'on','on','on','on','off','off','on',get_param(gcb,'PlotResponse')};end;set_param(gcb,'MaskVisibilities',visible)|||p7=get_param(gcb,'PlotResponse');if strcmp(p7,'on');visible={'on','on','on','on',get_param(gcb,'Initialize'),get_param(gcb,'Initialize'),'on','on'};else;visible={'on','on','on','on',get_param(gcb,'Initialize'),get_param(gcb,'Initialize'),'on','off'};end;set_param(gcb,'MaskVisibilities',visible)|
      mask Display: plot(X,Y);
  VS : Outport  InitialOutput=0
  wires:
  Lead-Lag #1/1(Out1) -> Lead-Lag #2/1(In1)
  In/1 -> "Sensor "/1(In)
  "Sensor "/1(Out) -> Overall Gain/1
  Overall Gain/1 -> "Wash-out "/1(In)
  "Wash-out "/1(Out) -> Lead-Lag #1/1(In1)
  Lead-Lag #2/1(Out1) -> "Limiter "/1
  "Limiter "/1 -> VS/1

== system powerlib_modelsV2/Discrete/Three-Level Bridge ==
  v : Inport  Port=1  PortDimensions=nb_arm*3  LatchInput=off
  g : Inport  Port=2  PortDimensions=nb_arm*4  LatchInput=off
  2-level GTO-IGBT Bridge  Logic (modified) : Subsystem  AncestorBlock=powerlib_models/Discrete/GTO-IGBT Bridge  mask(GTO & IGBT Bridge Logic(modified)){nb_arm=nb_arm, Tf=0, Tt=0, Cs=Cs, VFs=Par_Vf, Rsw=Ron, Ts=Ts}
      mask prompts: nb_arm "Number of bridge arms (1,2 or 3)"; Tf "Curent 10% fall time Tf (s) :"; Tt "Current tail time Tt (s) :"; Cs "Snubber Capacitance Cs (F):"; VFs "Forward Voltages [ Vf  Vfd ]"; Rsw "Device resistance"; Ts "Time step Ts (s) :"
      mask help:
      | Generates the switch status ( 0 or 1) and the tail currents for a forced-commutated two- level bridge using GTO/Diode or IGBT/Diode pairs.
      | Specify  3 arms (6 switches) for 3 phase bridge, 2 arms for 4 switches, or 1 arm.
      | To turn-off the tail current, specify Tf=0 and Tt=0.
      mask init: same as powerlib_modelsV2/Continuous/Three-Level Bridge/2-level GTO-IGBT Bridge  Logic (modified)
  Input : Subsystem
  Mux : Mux  Inputs=[nb_arm*2 nb_arm]
  Mux1 : Mux  Inputs=[nb_arm*2 nb_arm]
  Select_Status : Selector  Elements=StatusElements  InputPortWidth=3*nb_arm
  Select_Status1 : Selector  Elements=StatusElements  InputPortWidth=3*nb_arm
  SubSystem : Subsystem
      mask Display: disp('?')
  Sw3 (clamping diode) Logic : Subsystem  mask{nb_arm=nb_arm, VFs=Par_Vf, Ts=Ts}
      mask prompts: nb_arm "Number of bridge arm:"; VFs "Forward Voltages [ Vf  Vfd ]"; Ts "Sample time:"
      mask init: same as powerlib_modelsV2/Continuous/Three-Level Bridge/Sw3 (clamping diode) Logic
  x : Outport
  Status : Outport  Port=2
  Vf : Outport  Port=3
  wires:
  Select_Status1/1 -> Vf/1
  Select_Status/1 -> Status/1, x/1
  2-level GTO-IGBT Bridge  Logic (modified)/3(Block3) -> Sw3 (clamping diode) Logic/3(Block3)
  Sw3 (clamping diode) Logic/4(Block12) -> 2-level GTO-IGBT Bridge  Logic (modified)/3(Block12)
  Sw3 (clamping diode) Logic/3(g12) -> 2-level GTO-IGBT Bridge  Logic (modified)/2(g)
  Sw3 (clamping diode) Logic/2(Vf) -> Mux1/2
  Sw3 (clamping diode) Logic/1(Status) -> Mux/2
  2-level GTO-IGBT Bridge  Logic (modified)/2(Vf) -> Mux1/1
  Mux/1 -> Select_Status/1
  Mux1/1 -> Select_Status1/1
  2-level GTO-IGBT Bridge  Logic (modified)/1(status) -> Mux/1
  v/1 -> Sw3 (clamping diode) Logic/1(V_Sw123), 2-level GTO-IGBT Bridge  Logic (modified)/1(v)
  Sw3 (clamping diode) Logic/5(Trig12) -> 2-level GTO-IGBT Bridge  Logic (modified)/4(Trig12)
  g/1 -> Input/1(In)
  Input/1(Out) -> Sw3 (clamping diode) Logic/2(Pulses)
  2-level GTO-IGBT Bridge  Logic (modified)/4(status_GTO) -> Sw3 (clamping diode) Logic/4(Status_GTO)

== system powerlib_modelsV2/Discrete/asynchronous_machine ==
  v : Inport  Port=1  LatchInput=off
  Tm : Inport  Port=2  LatchInput=off
  Gain : Gain  Gain=[ib2*ones(5,1);phib2;phib2;Vb2;Vb2;ib2*ones(5,1);phib2;phib2;Vb2;Vb2;Nb2;Tb2;1]  SaturateOnIntegerOverflow=on
  Mechanical : Subsystem  Orientation=left
      mask Display: disp('Mechanical')
  Mutual fluxes : Subsystem  Orientation=left
  Mux3 : Mux  Inputs=[3,2,2,2,3,2,2,2,3]
  Rotor : Subsystem
      mask Display: disp('Rotor')
  Stator : Subsystem
      mask Display: disp('Stator')
  abc2qd : Subsystem
      mask Display: disp('abc2qd')
  dq2abc : Subsystem
  sin,cos : Subsystem
  i : Outport
  m : Outport  Port=2
  wires:
  sin,cos/2(w-wr) -> Rotor/2(w-wr)
  Mutual fluxes/1(phimq,phimd) -> Rotor/3(phimq,phimd), Stator/1(phimq,phimd)
  sin,cos/1(sin,cos) -> abc2qd/2(sin,cos), dq2abc/1(sin,cos)
  Stator/3(phis,is) -> Mechanical/2(phis,is)
  sin,cos/3(w) -> Stator/3(w)
  abc2qd/2(vqs,vds) -> Stator/2(vqs,vds), Mux3/8
  abc2qd/1(vqr,vdr) -> Rotor/1(vqr,vdr), Mux3/4
  dq2abc/1(irab,isab) -> i/1
  Rotor/2(phiqr,phidr) -> Mutual fluxes/1(phiqr,phidr), Mux3/3
  Rotor/1(iqr,idr) -> Mux3/2, dq2abc/2(iqr,idr)
  v/1 -> abc2qd/1(v)
  Mechanical/2(thr,wr) -> sin,cos/1(thr,wr)
  Stator/1(phiqs,phids) -> Mutual fluxes/2(phiqs,phids), Mux3/7
  Stator/2(iqs,ids) -> dq2abc/3(iqs,ids), Mux3/6
  Mechanical/1(w,Te,thr) -> Mux3/9
  Mux3/1 -> Gain/1
  Gain/1 -> m/1
  dq2abc/3(isabc) -> Mux3/5
  dq2abc/2(irabc) -> Mux3/1
  Tm/1 -> Mechanical/1(Tm)

== system powerlib_modelsV2/Discrete/breaker ==
  note: Zero crossing detection
  note: Current Prediction
  v : Inport  Port=1  LatchInput=off
  g : Inport  Port=2  LatchInput=off
  0 1 : Constant  Value=0
  >1.5 : Relay  OnSwitchValue=1.5  OffSwitchValue=0
  Constant : Constant  Value=zeros(Nsw,1)
  Data Type  Conversion{,1..3} (4 alike) : DataTypeConversion  SaturateOnIntegerOverflow=on  RndMeth=Zero
  Data Type  Conversion4 : DataTypeConversion  Orientation=up  SaturateOnIntegerOverflow=on  RndMeth=Zero
  Delay Ts : UnitDelay  SampleTime=Ts
  "Delay Ts " : UnitDelay  SampleTime=Ts
  Delay Ts 1 : UnitDelay  SampleTime=Ts
  Gain : Gain  Gain=2  SaturateOnIntegerOverflow=on
  IC : InitialCondition  Value=istate
  Product : Product  SaturateOnIntegerOverflow=on  InputSameDT=on
  Sum : Sum  Inputs=+-  SaturateOnIntegerOverflow=on  InputSameDT=on
  b5 : RelationalOperator  Operator=>  InputSameDT=on
  or : Logic  Operator=OR
  sum : Sum  SaturateOnIntegerOverflow=on  InputSameDT=on
  i : Outport  InitialOutput=0
  Status : Outport  Port=2  InitialOutput=0
  wires:
  Data Type  Conversion4/1 -> sum/2
  Product/1 -> b5/1
  b5/1 -> Data Type  Conversion2/1
  Data Type  Conversion/1 -> IC/1
  or/1 -> Data Type  Conversion/1
  IC/1 -> Status/1
  Data Type  Conversion1/1 -> or/1
  Delay Ts 1/1 -> Data Type  Conversion1/1
  Data Type  Conversion3/1 -> or/2
  >1.5/1 -> Delay Ts 1/1
  g/1 -> Data Type  Conversion4/1, Data Type  Conversion3/1
  Constant/1 -> i/1
  sum/1 -> >1.5/1
  Data Type  Conversion2/1 -> sum/1
  0 1/1 -> b5/2
  "Delay Ts "/1 -> Product/2
  Sum/1 -> "Delay Ts "/1, Product/1
  v/1 -> Delay Ts/1, Gain/1  "Braeker voltage"
  Delay Ts/1 -> Sum/2
  Gain/1 -> Sum/1

== system powerlib_modelsV2/Discrete/detailed_thyristor (logical) ==
  note: Current prediction
  v : Inport  Port=1  LatchInput=off
  g : Inport  Port=2  LatchInput=off
  " Delay Ts1" : UnitDelay  SampleTime=Ts
  " Delay Ts2" : UnitDelay  SampleTime=Ts
  0 {1..4} (4 alike) : Constant  Value=0
  1/Rsw : Gain  Gain=1/Rsw  SaturateOnIntegerOverflow=on
  Constant : Constant  Value=zeros(Nsw,1)
  Data Type  Conversion{1..5} (5 alike) : DataTypeConversion  SaturateOnIntegerOverflow=on  RndMeth=Zero
  Gain : Gain  Gain=2  SaturateOnIntegerOverflow=on
  Mux : Mux  Inputs=2
  Saturation : Saturate  UpperLimit=inf  LowerLimit=0
  Sum : Sum  Inputs=+-  SaturateOnIntegerOverflow=on  InputSameDT=on
  Sum1 : Sum  Inputs=|++  SaturateOnIntegerOverflow=on  InputSameDT=on
  Switch : Switch  Threshold=0.5  InputSameDT=on
  b5 : RelationalOperator  Operator=>  InputSameDT=on
  b6 : RelationalOperator  Operator=>  InputSameDT=on
  b7 : RelationalOperator  Operator===  InputSameDT=on
  or2 : Logic  Operator=OR
  or3 : Logic  Inputs=3
  vf : Constant  Value=Vf
  i : Outport  InitialOutput=0
  Status : Outport  Port=2  InitialOutput=0
  m : Outport  Port=3  InitialOutput=0
  Vf : Outport  Port=4  InitialOutput=0
  wires:
  0 3/1 -> b7/2
  v/1 -> b6/1, Sum1/1, 1/Rsw/1  "Vak"
  0 2/1 -> b6/2
  Gain/1 -> Sum/1
  " Delay Ts1"/1 -> Sum/2
  0 1/1 -> b5/2
  Sum/1 -> b5/1
  or3/1 -> or2/2
  Mux/1 -> m/1  "measurement signals"
  Constant/1 -> i/1
  Sum1/1 -> Mux/2
  vf/1 -> Sum1/2, Vf/1
  or2/1 -> Data Type  Conversion1/1
  Data Type  Conversion1/1 -> " Delay Ts2"/1
  " Delay Ts2"/1 -> Status/1, Switch/2
  g/1 -> Data Type  Conversion2/1
  Data Type  Conversion2/1 -> or3/2
  b7/1 -> Data Type  Conversion3/1
  Data Type  Conversion3/1 -> or3/3
  b6/1 -> Data Type  Conversion4/1
  Data Type  Conversion4/1 -> or3/1
  b5/1 -> Data Type  Conversion5/1
  Data Type  Conversion5/1 -> or2/1
  Switch/1 -> Saturation/1
  Saturation/1 -> Mux/1, b7/1, Gain/1, " Delay Ts1"/1
  1/Rsw/1 -> Switch/1  "Iak"
  0 4/1 -> Switch/3

== system powerlib_modelsV2/Discrete/diode (logical) ==
  note: Current Prediction
  v : Inport  Port=1  LatchInput=off
  " Delay Ts" : UnitDelay  SampleTime=Ts
  " Delay Ts1" : UnitDelay  SampleTime=Ts
  0 {1..4} (4 alike) : Constant  Value=0
  1/Rsw : Gain  Gain=1./Rsw  SaturateOnIntegerOverflow=on
  Constant : Constant  Value=zeros(Nsw,1)
  Data Type  Conversion1 : DataTypeConversion  SaturateOnIntegerOverflow=on  RndMeth=Zero
  Gain : Gain  Gain=2  SaturateOnIntegerOverflow=on
  Mux : Mux  Inputs=2
  Saturation : Saturate  UpperLimit=inf  LowerLimit=0
  Sum : Sum  Inputs=+-  SaturateOnIntegerOverflow=on  InputSameDT=on
  Sum1 : Sum  Inputs=|++  SaturateOnIntegerOverflow=on  InputSameDT=on
  Switch : Switch  Threshold=0.5  InputSameDT=on
  b5 : RelationalOperator  Operator=>  InputSameDT=on
  b6 : RelationalOperator  Operator=>  InputSameDT=on
  b7 : RelationalOperator  Operator===  InputSameDT=on
  or2 : Logic  Operator=OR
  or3 : Logic
  vf : Constant  Value=Vf
  i : Outport  InitialOutput=0
  Status : Outport  Port=2  InitialOutput=0
  m : Outport  Port=3  InitialOutput=0
  Vf : Outport  Port=4  InitialOutput=0
  wires:
  Mux/1 -> m/1  "measurement signals"
  b5/1 -> or2/1
  Sum/1 -> b5/1
  0 1/1 -> b5/2
  " Delay Ts"/1 -> Sum/2
  Gain/1 -> Sum/1
  0 2/1 -> b6/2
  v/1 -> b6/1, Sum1/1, 1/Rsw/1  "Vak"
  0 3/1 -> b7/2
  or3/1 -> or2/2
  b6/1 -> or3/1
  b7/1 -> or3/2
  Constant/1 -> i/1
  Sum1/1 -> Mux/2
  vf/1 -> Sum1/2, Vf/1
  or2/1 -> Data Type  Conversion1/1
  Data Type  Conversion1/1 -> " Delay Ts1"/1
  " Delay Ts1"/1 -> Status/1, Switch/2
  1/Rsw/1 -> Switch/1  "Iak"
  Switch/1 -> Saturation/1
  Saturation/1 -> Mux/1, b7/1, Gain/1, " Delay Ts"/1
  0 4/1 -> Switch/3
